simulink model "prescan_repl_stopCriteria"  (R2019a)
settings: Solver=VariableStepAuto  StartTime=0.0  StopTime=1000  RelTol=1e-3
libraries: ProSivic_Sensors x2, realtime_pacer_lib x1
settings Model: Creator=Markus Borg  LastModifiedBy=Markus Borg

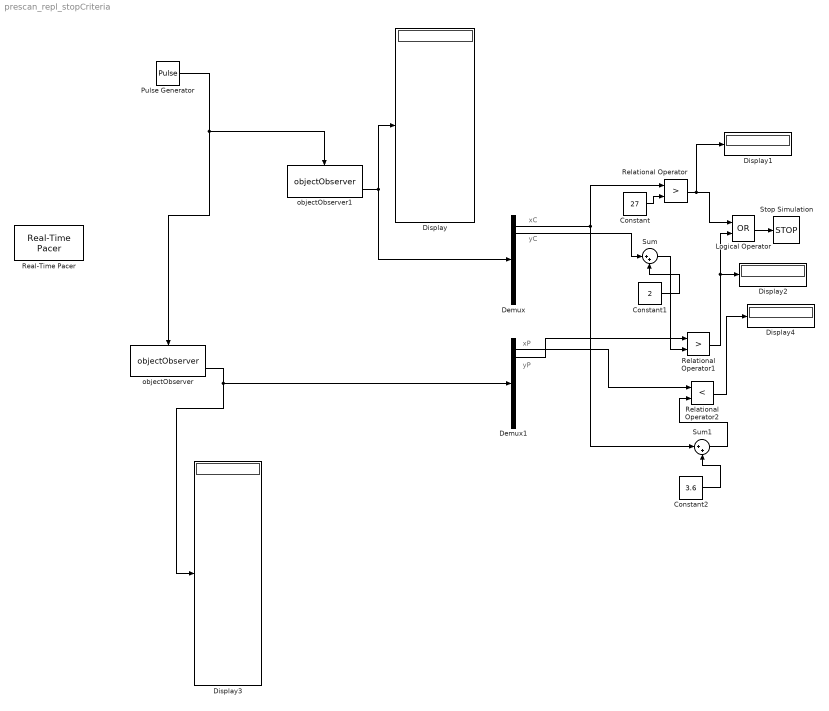
== system prescan_repl_stopCriteria ==
  note: yP
  note: yC
  note: xP
  note: xC
  Constant : Constant  Value=27
  Constant1 : Constant  Value=2
  Constant2 : Constant  Value=3.6
  Demux : Demux  Outputs=10
  Demux1 : Demux  Outputs=10
  Display{,1..4} (5 alike) : Display
  Logical Operator : Logic  Operator=OR  AllPortsSameDT=off  OutDataTypeStr=boolean
  Pulse Generator : DiscretePulseGenerator  PulseType=Time based  Period=0.5  PulseWidth=50
  Real-Time Pacer : realtime_pacer_lib/Real-Time Pacer  simTimePerRealTime=10
  Relational Operator : RelationalOperator  Operator=>  OutDataTypeStr=boolean  RndMeth=Simplest
  Relational Operator1 : RelationalOperator  Operator=>  OutDataTypeStr=boolean  RndMeth=Simplest
  Relational Operator2 : RelationalOperator  Operator=<  OutDataTypeStr=boolean  RndMeth=Simplest
  Stop Simulation : Stop
  Sum : Sum  Inputs=|++
  Sum1 : Sum  Inputs=|++
  objectObserver : ProSivic_Sensors/objectObserver  topic=ped_obs
  objectObserver1 : ProSivic_Sensors/objectObserver  topic=car_obs
  wires:
  Pulse Generator/1 -> objectObserver1/Trigger, objectObserver/Trigger
  Relational Operator1/1 -> Display2/1, Logical Operator/2
  Demux1/1 -> Relational Operator2/1
  Constant/1 -> Relational Operator/2
  Relational Operator2/1 -> Display4/1
  objectObserver/2 -> Demux1/1, Display3/1
  Relational Operator/1 -> Display1/1, Logical Operator/1
  Constant1/1 -> Sum/2
  Demux1/2 -> Relational Operator1/1
  Constant2/1 -> Sum1/2
  objectObserver1/2 -> Demux/1, Display/1
  Demux/1 -> Relational Operator/1, Sum1/1
  Sum1/1 -> Relational Operator2/2
  Sum/1 -> Relational Operator1/2
  Demux/2 -> Sum/1
  Logical Operator/1 -> Stop Simulation/1
